simulink model "Desorbtion_mass_1604"  (Simulink 7.7)
settings: Solver=ode23tb  StartTime=0.0  StopTime=7000  FixedStep=0.01  RelTol=1e-3
libraries: simulink x2
settings Model: Creator=User  LastModifiedBy=Natalia
settings OptimizationCC: InitFltsAndDblsToZero=on
settings DebuggingCC: StrictBusMsg=Warning

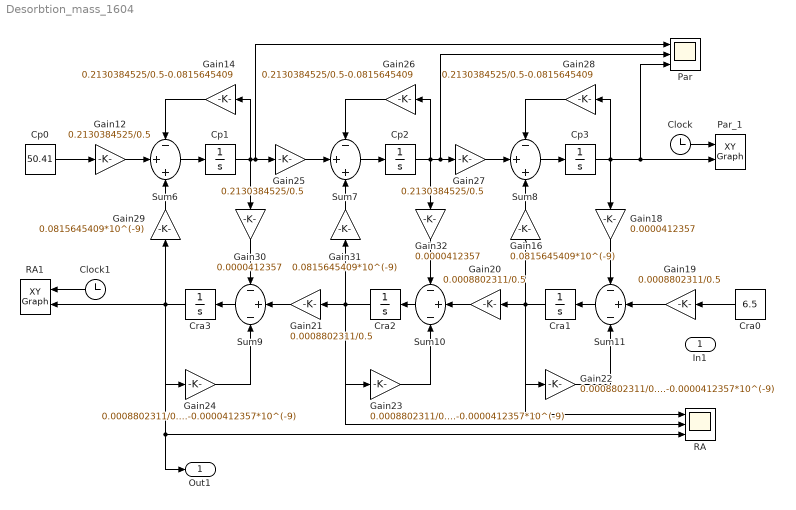
== system Desorbtion_mass_1604 ==
  In1 : Inport
  Clock : Clock
      settings: Decimation=10800
  Clock1 : Clock
      settings: Decimation=10800
  Cp0 : Constant  Value=50.41
  Cp1 : Integrator  InitialCondition=62.344748750140901
  Cp2 : Integrator  InitialCondition=77.105092178789903
  Cp3 : Integrator  InitialCondition=95.359999985633294
  Cra0 : Constant  Value=6.5
  Cra1 : Integrator  InitialCondition=4.266361384395665
  Cra2 : Integrator  InitialCondition=2.460311558699043
  Cra3 : Integrator  InitialCondition=0.999996559606798
  Gain12 : Gain  Gain=0.2130384525/0.5
  Gain14 : Gain  Gain=0.2130384525/0.5-0.0815645409
  Gain16 : Gain  Gain=0.0815645409*10^(-9)
  Gain18 : Gain  Gain=0.0000412357
  Gain19 : Gain  Gain=0.0008802311/0.5
  Gain20 : Gain  Gain=0.0008802311/0.5
  Gain21 : Gain  Gain=0.0008802311/0.5
  Gain22 : Gain  Gain=0.0008802311/0.5-0.0000412357*10^(-9)
  Gain23 : Gain  Gain=0.0008802311/0.5-0.0000412357*10^(-9)
  Gain24 : Gain  Gain=0.0008802311/0.5-0.0000412357*10^(-9)
  Gain25 : Gain  Gain=0.2130384525/0.5
  Gain26 : Gain  Gain=0.2130384525/0.5-0.0815645409
  Gain27 : Gain  Gain=0.2130384525/0.5
  Gain28 : Gain  Gain=0.2130384525/0.5-0.0815645409
  Gain29 : Gain  Gain=0.0815645409*10^(-9)
  Gain30 : Gain  Gain=0.0000412357
  Gain31 : Gain  Gain=0.0815645409*10^(-9)
  Gain32 : Gain  Gain=0.0000412357
  Par : Scope  NumInputPorts=3
      settings: TimeRange=12  YMin=62.3447~77.1051~95.36  YMax=62.3447~77.1051~95.36
  Par_1 : simulink/Sinks/XY Graph  SystemSampleTime=-1  xmin=0  xmax=7000  ymin=95  ymax=96  st=-1
  RA : Scope  NumInputPorts=3
      settings: YMin=4.26636~2.46031~1  YMax=4.26636~2.46031~1
  RA1 : simulink/Sinks/XY Graph  SystemSampleTime=-1  xmin=0  xmax=7000  ymin=0  ymax=2  st=-1
  Sum10 : Sum  Inputs=-+-
  Sum11 : Sum  Inputs=-+-
  Sum6 : Sum  Inputs=-++
  Sum7 : Sum  Inputs=-++
  Sum8 : Sum  Inputs=-++
  Sum9 : Sum  Inputs=-+-
  Out1 : Outport
  wires:
  Gain12/1 -> Sum6/2
  Gain14/1 -> Sum6/1
  Sum6/1 -> Cp1/1
  Gain25/1 -> Sum7/2
  Gain26/1 -> Sum7/1
  Sum7/1 -> Cp2/1
  Gain27/1 -> Sum8/2
  Gain28/1 -> Sum8/1
  Sum8/1 -> Cp3/1
  Cp1/1 -> Gain30/1, Gain14/1, Gain25/1, Par/1
  Cp2/1 -> Gain32/1, Gain26/1, Gain27/1, Par/2
  Gain29/1 -> Sum6/3
  Cp3/1 -> Gain18/1, Gain28/1, Par_1/2, Par/3
  Gain31/1 -> Sum7/3
  Gain16/1 -> Sum8/3
  Clock/1 -> Par_1/1
  Gain30/1 -> Sum9/1
  Gain32/1 -> Sum10/1
  Gain18/1 -> Sum11/1
  Gain19/1 -> Sum11/2
  Sum11/1 -> Cra1/1
  Cra1/1 -> Gain16/1, Gain22/1, Gain20/1, RA/1
  Gain20/1 -> Sum10/2
  Sum10/1 -> Cra2/1
  Cra2/1 -> Gain31/1, Gain23/1, Gain21/1, RA/2
  Gain21/1 -> Sum9/2
  Sum9/1 -> Cra3/1
  Cra3/1 -> Gain29/1, Gain24/1, RA1/2, RA/3, Out1/1
  Gain22/1 -> Sum11/3
  Gain23/1 -> Sum10/3
  Gain24/1 -> Sum9/3
  Clock1/1 -> RA1/1
  Cp0/1 -> Gain12/1
  Cra0/1 -> Gain19/1
